simulink model "platforma3a"  (Simulink 8.3)
settings: Solver=ode23  StartTime=0.0  StopTime=80  RelTol=1e-8
values from neighbouring files (symbols this model uses):
  a = 0.365    [REX.m]
  b = 0.365    [REX.m]
  c = 0.387    [REX.m]
  d = 0.387    [REX.m]
  fr = 0    [REX.m]
  g = 9.81    [REX.m]
  Ik = 0.15    [REX.m]
  Ip = I    (= 6)    [REX.m]
  k1 = 1    [REX.m]
  k2 = 1    [REX.m]
  Kd = 500    [REX.m]
  mi = 0    [REX.m]
  mp = 40    [REX.m]
  omega = 0.1    [REX.m]
  R = 10    [REX.m]
  r = 0.127    [REX.m]
  tt = 0.387    [REX.m]
settings Model: Creator=mat  LastModifiedBy=Student
settings OptimizationCC: ExpressionDepthLimit=2147483647
settings DebuggingCC: FcnCallInpInsideContextMsg=UseLocalSettings

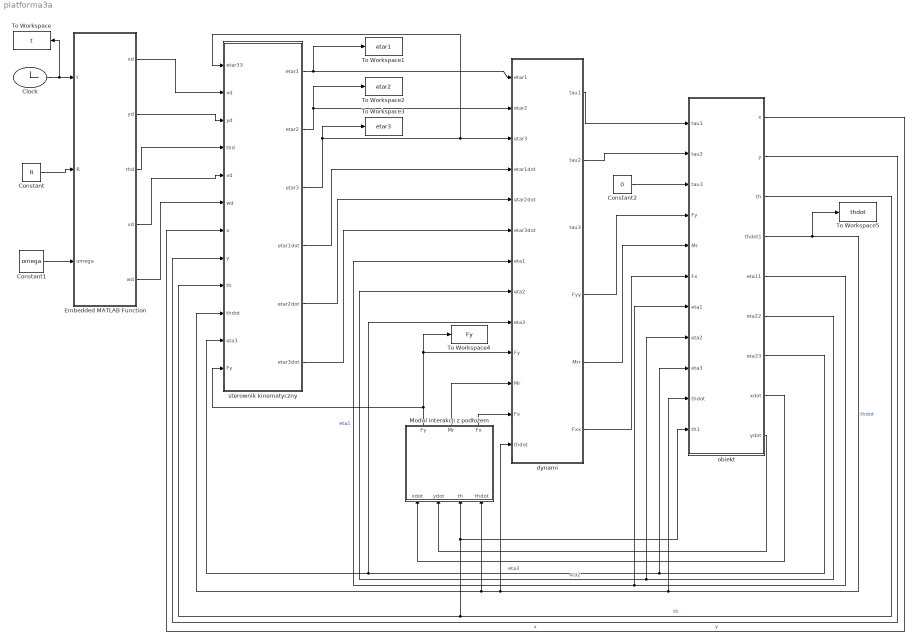
== system platforma3a ==
  Clock : Clock
  Constant : Constant  Value=R
  Constant1 : Constant  Value=omega
  Constant2 : Constant  Value=0
  Embedded MATLAB Function : MATLAB Function  TreatAsAtomicUnit=on
  Modul interakcji z podłożem : Subsystem
  To Workspace : ToWorkspace  VariableName=t  SampleTime=-1
  To Workspace1 : ToWorkspace  VariableName=etar1  SampleTime=-1
  To Workspace2 : ToWorkspace  VariableName=etar2  SampleTime=-1
  To Workspace3 : ToWorkspace  VariableName=etar3  SampleTime=-1
  To Workspace4 : ToWorkspace  VariableName=Fy  SampleTime=-1
  To Workspace5 : ToWorkspace  VariableName=thdot  SampleTime=-1
  dynami : Subsystem
  obiekt : Subsystem
  sterownik kinematyczny : Subsystem
  wires:
  Clock/1 -> Embedded MATLAB Function/1(t), To Workspace/1
  Constant/1 -> Embedded MATLAB Function/2(R)
  Constant1/1 -> Embedded MATLAB Function/3(omega)
  dynami/1(tau1) -> obiekt/1(tau1)
  dynami/2(tau2) -> obiekt/2(tau2)
  Modul interakcji z podłożem/3(Fx) -> dynami/12(Fx)
  dynami/4(Fyy) -> obiekt/4(Fy)
  dynami/5(Mrr) -> obiekt/5(Mr)
  dynami/6(Fxx) -> obiekt/6(Fx)
  obiekt/7(eta33) -> obiekt/9(eta3), dynami/9(eta3), sterownik kinematyczny/11(eta3)  "eta3"
  obiekt/6(eta22) -> obiekt/8(eta2), dynami/8(eta2)  "eta2"
  obiekt/5(eta11) -> obiekt/7(eta1), dynami/7(eta1)  "eta1"
  Embedded MATLAB Function/1(xd) -> sterownik kinematyczny/2(xd)
  Embedded MATLAB Function/2(yd) -> sterownik kinematyczny/3(yd)
  Embedded MATLAB Function/4(vd) -> sterownik kinematyczny/5(vd)
  Embedded MATLAB Function/5(wd) -> sterownik kinematyczny/6(wd)
  sterownik kinematyczny/1(etar1) -> dynami/1(etar1), To Workspace1/1
  sterownik kinematyczny/2(etar2) -> dynami/2(etar2), To Workspace2/1
  sterownik kinematyczny/3(etar3) -> To Workspace3/1, dynami/3(etar3), sterownik kinematyczny/1(etar33)
  sterownik kinematyczny/4(etar1dot) -> dynami/4(etar1dot)
  sterownik kinematyczny/5(etar2dot) -> dynami/5(etar2dot)
  sterownik kinematyczny/6(etar3dot) -> dynami/6(etar3dot)
  Modul interakcji z podłożem/2(Mr) -> dynami/11(Mr)
  Modul interakcji z podłożem/1(Fy) -> sterownik kinematyczny/12(Fy), dynami/10(Fy), To Workspace4/1
  obiekt/1(x) -> sterownik kinematyczny/7(x)  "x"
  obiekt/2(y) -> sterownik kinematyczny/8(y)  "y"
  obiekt/3(th) -> sterownik kinematyczny/9(th), Modul interakcji z podłożem/3(th), obiekt/11(th1)  "th"
  obiekt/4(thdot1) -> dynami/13(thdot), Modul interakcji z podłożem/4(thdot), sterownik kinematyczny/10(thdot), obiekt/10(thdot), To Workspace5/1  "thdot"
  obiekt/9(ydot) -> Modul interakcji z podłożem/2(ydot)
  obiekt/8(xdot) -> Modul interakcji z podłożem/1(xdot)
  Embedded MATLAB Function/3(thd) -> sterownik kinematyczny/4(thd)
  Constant2/1 -> obiekt/3(tau3)

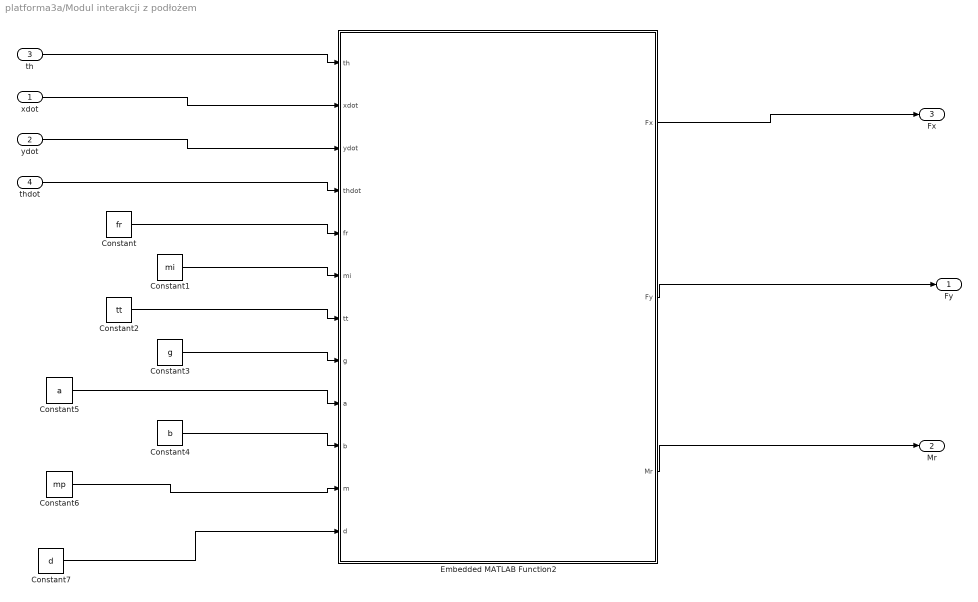
== system platforma3a/Modul interakcji z podłożem ==
  xdot : Inport
  ydot : Inport  Port=2
  th : Inport  Port=3
  thdot : Inport  Port=4
  Constant : Constant  Value=fr
  Constant1 : Constant  Value=mi
  Constant2 : Constant  Value=tt
  Constant3 : Constant  Value=g
  Constant4 : Constant  Value=b
  Constant5 : Constant  Value=a
  Constant6 : Constant  Value=mp
  Constant7 : Constant  Value=d
  Embedded MATLAB Function2 : MATLAB Function  TreatAsAtomicUnit=on
  Fy : Outport
  Mr : Outport  Port=2
  Fx : Outport  Port=3
  wires:
  th/1 -> Embedded MATLAB Function2/1(th)
  thdot/1 -> Embedded MATLAB Function2/4(thdot)
  Constant/1 -> Embedded MATLAB Function2/5(fr)
  Constant1/1 -> Embedded MATLAB Function2/6(mi)
  Constant2/1 -> Embedded MATLAB Function2/7(tt)
  Constant3/1 -> Embedded MATLAB Function2/8(g)
  Constant5/1 -> Embedded MATLAB Function2/9(a)
  Constant4/1 -> Embedded MATLAB Function2/10(b)
  Constant6/1 -> Embedded MATLAB Function2/11(m)
  Constant7/1 -> Embedded MATLAB Function2/12(d)
  Embedded MATLAB Function2/3(Mr) -> Mr/1
  Embedded MATLAB Function2/2(Fy) -> Fy/1
  Embedded MATLAB Function2/1(Fx) -> Fx/1
  xdot/1 -> Embedded MATLAB Function2/2(xdot)
  ydot/1 -> Embedded MATLAB Function2/3(ydot)

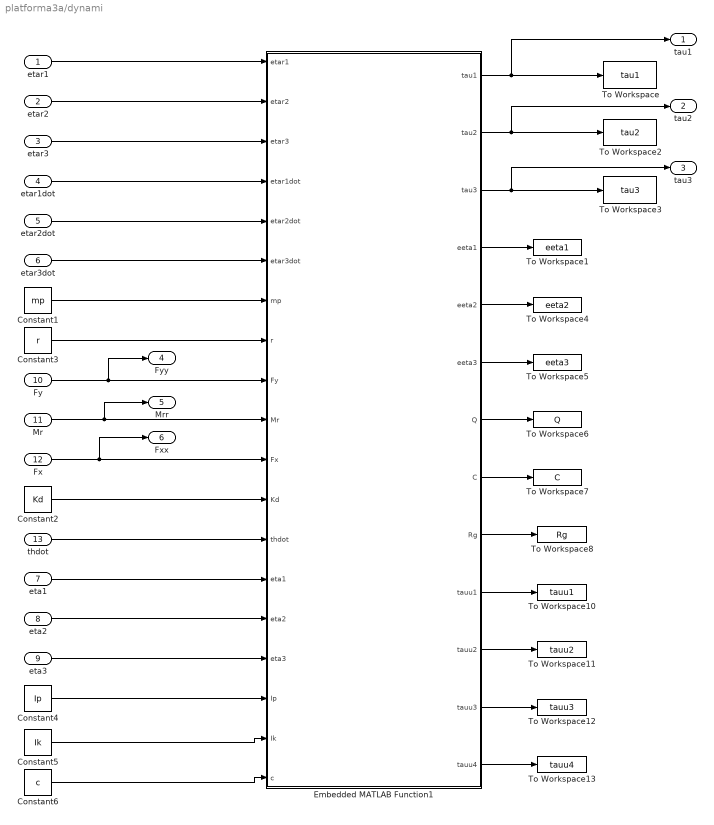
== system platforma3a/dynami ==
  etar1 : Inport
  etar2 : Inport  Port=2
  etar3 : Inport  Port=3
  etar1dot : Inport  Port=4
  etar2dot : Inport  Port=5
  etar3dot : Inport  Port=6
  eta1 : Inport  Port=7
  eta2 : Inport  Port=8
  eta3 : Inport  Port=9
  Fy : Inport  Port=10
  Mr : Inport  Port=11
  Fx : Inport  Port=12
  thdot : Inport  Port=13
  Constant1 : Constant  Value=mp
  Constant2 : Constant  Value=Kd
  Constant3 : Constant  Value=r
  Constant4 : Constant  Value=Ip
  Constant5 : Constant  Value=Ik
  Constant6 : Constant  Value=c
  Embedded MATLAB Function1 : MATLAB Function  TreatAsAtomicUnit=on
  To Workspace : ToWorkspace  VariableName=tau1  SampleTime=-1
  To Workspace1 : ToWorkspace  VariableName=eeta1  SampleTime=-1
  To Workspace10 : ToWorkspace  VariableName=tauu1  SampleTime=-1
  To Workspace11 : ToWorkspace  VariableName=tauu2  SampleTime=-1
  To Workspace12 : ToWorkspace  VariableName=tauu3  SampleTime=-1
  To Workspace13 : ToWorkspace  VariableName=tauu4  SampleTime=-1
  To Workspace2 : ToWorkspace  VariableName=tau2  SampleTime=-1
  To Workspace3 : ToWorkspace  VariableName=tau3  SampleTime=-1
  To Workspace4 : ToWorkspace  VariableName=eeta2  SampleTime=-1
  To Workspace5 : ToWorkspace  VariableName=eeta3  SampleTime=-1
  To Workspace6 : ToWorkspace  VariableName=Q  SampleTime=-1
  To Workspace7 : ToWorkspace  VariableName=C  SampleTime=-1
  To Workspace8 : ToWorkspace  VariableName=Rg  SampleTime=-1
  tau1 : Outport
  tau2 : Outport  Port=2
  tau3 : Outport  Port=3
  Fyy : Outport  Port=4
  Mrr : Outport  Port=5
  Fxx : Outport  Port=6
  wires:
  etar1/1 -> Embedded MATLAB Function1/1(etar1)
  etar2/1 -> Embedded MATLAB Function1/2(etar2)
  Embedded MATLAB Function1/1(tau1) -> tau1/1, To Workspace/1
  Embedded MATLAB Function1/2(tau2) -> To Workspace2/1, tau2/1
  Embedded MATLAB Function1/6(eeta3) -> To Workspace5/1
  Embedded MATLAB Function1/4(eeta1) -> To Workspace1/1
  Embedded MATLAB Function1/5(eeta2) -> To Workspace4/1
  Embedded MATLAB Function1/7(Q) -> To Workspace6/1
  Embedded MATLAB Function1/8(C) -> To Workspace7/1
  Embedded MATLAB Function1/9(Rg) -> To Workspace8/1
  Constant5/1 -> Embedded MATLAB Function1/18(Ik)
  Constant4/1 -> Embedded MATLAB Function1/17(Ip)
  eta3/1 -> Embedded MATLAB Function1/16(eta3)
  eta2/1 -> Embedded MATLAB Function1/15(eta2)
  eta1/1 -> Embedded MATLAB Function1/14(eta1)
  thdot/1 -> Embedded MATLAB Function1/13(thdot)
  Constant2/1 -> Embedded MATLAB Function1/12(Kd)
  Constant3/1 -> Embedded MATLAB Function1/8(r)
  Constant1/1 -> Embedded MATLAB Function1/7(mp)
  etar3dot/1 -> Embedded MATLAB Function1/6(etar3dot)
  etar2dot/1 -> Embedded MATLAB Function1/5(etar2dot)
  etar1dot/1 -> Embedded MATLAB Function1/4(etar1dot)
  etar3/1 -> Embedded MATLAB Function1/3(etar3)
  Embedded MATLAB Function1/13(tauu4) -> To Workspace13/1
  Embedded MATLAB Function1/12(tauu3) -> To Workspace12/1
  Embedded MATLAB Function1/11(tauu2) -> To Workspace11/1
  Embedded MATLAB Function1/10(tauu1) -> To Workspace10/1
  Constant6/1 -> Embedded MATLAB Function1/19(c)
  Fy/1 -> Embedded MATLAB Function1/9(Fy), Fyy/1
  Mr/1 -> Embedded MATLAB Function1/10(Mr), Mrr/1
  Fx/1 -> Embedded MATLAB Function1/11(Fx), Fxx/1
  Embedded MATLAB Function1/3(tau3) -> To Workspace3/1, tau3/1

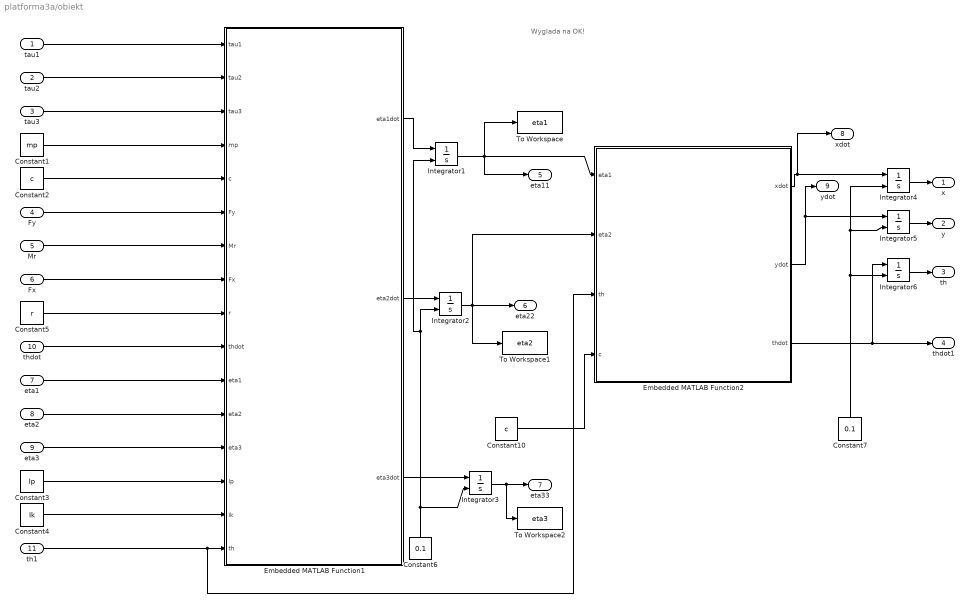
== system platforma3a/obiekt ==
  note: Wyglada na OK!
  tau1 : Inport
  tau2 : Inport  Port=2
  tau3 : Inport  Port=3
  Fy : Inport  Port=4
  Mr : Inport  Port=5
  Fx : Inport  Port=6
  eta1 : Inport  Port=7
  eta2 : Inport  Port=8
  eta3 : Inport  Port=9
  thdot : Inport  Port=10
  th1 : Inport  Port=11
  Constant1 : Constant  Value=mp
  Constant10 : Constant  Value=c
  Constant2 : Constant  Value=c
  Constant3 : Constant  Value=Ip
  Constant4 : Constant  Value=Ik
  Constant5 : Constant  Value=r
  Constant6 : Constant  Value=0.1
  Constant7 : Constant  Value=0.1
  Embedded MATLAB Function1 : MATLAB Function  TreatAsAtomicUnit=on
  Embedded MATLAB Function2 : MATLAB Function  TreatAsAtomicUnit=on
  Integrator{1..6} (6 alike) : Integrator  InitialConditionSource=external
  To Workspace : ToWorkspace  VariableName=eta1  SampleTime=-1
  To Workspace1 : ToWorkspace  VariableName=eta2  SampleTime=-1
  To Workspace2 : ToWorkspace  VariableName=eta3  SampleTime=-1
  x : Outport
  y : Outport  Port=2
  th : Outport  Port=3
  thdot1 : Outport  Port=4
  eta11 : Outport  Port=5
  eta22 : Outport  Port=6
  eta33 : Outport  Port=7
  xdot : Outport  Port=8
  ydot : Outport  Port=9
  wires:
  Constant1/1 -> Embedded MATLAB Function1/4(mp)
  Fy/1 -> Embedded MATLAB Function1/6(Fy)
  Mr/1 -> Embedded MATLAB Function1/7(Mr)
  tau1/1 -> Embedded MATLAB Function1/1(tau1)
  tau3/1 -> Embedded MATLAB Function1/3(tau3)
  tau2/1 -> Embedded MATLAB Function1/2(tau2)
  eta3/1 -> Embedded MATLAB Function1/13(eta3)
  eta1/1 -> Embedded MATLAB Function1/11(eta1)
  eta2/1 -> Embedded MATLAB Function1/12(eta2)
  thdot/1 -> Embedded MATLAB Function1/10(thdot)
  Fx/1 -> Embedded MATLAB Function1/8(Fx)
  Constant5/1 -> Embedded MATLAB Function1/9(r)
  Embedded MATLAB Function1/3(eta3dot) -> Integrator3/1
  Embedded MATLAB Function1/2(eta2dot) -> Integrator2/1
  Embedded MATLAB Function1/1(eta1dot) -> Integrator1/1
  Constant2/1 -> Embedded MATLAB Function1/5(c)
  Constant3/1 -> Embedded MATLAB Function1/14(Ip)
  Constant4/1 -> Embedded MATLAB Function1/15(Ik)
  Constant6/1 -> Integrator1/2, Integrator2/2, Integrator3/2
  Integrator3/1 -> eta33/1, To Workspace2/1
  Embedded MATLAB Function2/1(xdot) -> Integrator4/1, xdot/1
  Integrator4/1 -> x/1
  Integrator5/1 -> y/1
  Embedded MATLAB Function2/2(ydot) -> Integrator5/1, ydot/1
  Integrator6/1 -> th/1
  Constant7/1 -> Integrator4/2, Integrator5/2, Integrator6/2
  th1/1 -> Embedded MATLAB Function1/16(th), Embedded MATLAB Function2/3(th)
  Integrator1/1 -> To Workspace/1, eta11/1, Embedded MATLAB Function2/1(eta1)
  Integrator2/1 -> To Workspace1/1, Embedded MATLAB Function2/2(eta2), eta22/1
  Constant10/1 -> Embedded MATLAB Function2/4(c)
  Embedded MATLAB Function2/3(thdot) -> thdot1/1, Integrator6/1

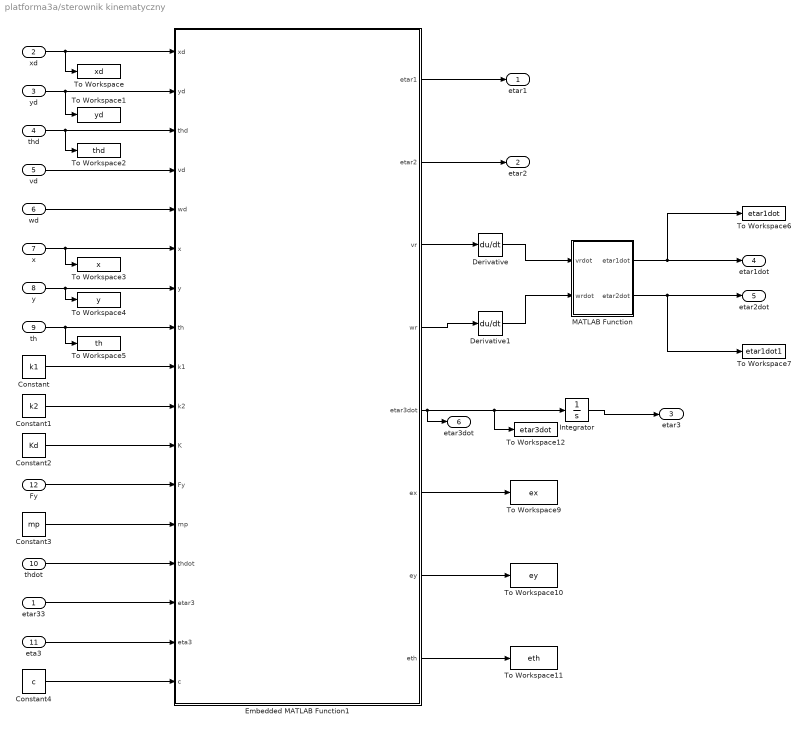
== system platforma3a/sterownik kinematyczny ==
  etar33 : Inport
  xd : Inport  Port=2
  yd : Inport  Port=3
  thd : Inport  Port=4
  vd : Inport  Port=5
  wd : Inport  Port=6
  x : Inport  Port=7
  y : Inport  Port=8
  th : Inport  Port=9
  thdot : Inport  Port=10
  eta3 : Inport  Port=11
  Fy : Inport  Port=12
  Constant : Constant  Value=k1
  Constant1 : Constant  Value=k2
  Constant2 : Constant  Value=Kd
  Constant3 : Constant  Value=mp
  Constant4 : Constant  Value=c
  Derivative : Derivative
  Derivative1 : Derivative
  Embedded MATLAB Function1 : MATLAB Function  TreatAsAtomicUnit=on
  Integrator : Integrator  InitialCondition=0.1
  MATLAB Function : MATLAB Function  TreatAsAtomicUnit=on
  To Workspace : ToWorkspace  VariableName=xd  SampleTime=-1
  To Workspace1 : ToWorkspace  VariableName=yd  SampleTime=-1
  To Workspace10 : ToWorkspace  VariableName=ey  SampleTime=-1
  To Workspace11 : ToWorkspace  VariableName=eth  SampleTime=-1
  To Workspace12 : ToWorkspace  VariableName=etar3dot  SampleTime=-1
  To Workspace2 : ToWorkspace  VariableName=thd  SampleTime=-1
  To Workspace3 : ToWorkspace  VariableName=x  SampleTime=-1
  To Workspace4 : ToWorkspace  VariableName=y  SampleTime=-1
  To Workspace5 : ToWorkspace  VariableName=th  SampleTime=-1
  To Workspace6 : ToWorkspace  VariableName=etar1dot  SampleTime=-1
  To Workspace7 : ToWorkspace  VariableName=etar1dot1  SampleTime=-1
  To Workspace9 : ToWorkspace  VariableName=ex  SampleTime=-1
  etar1 : Outport
  etar2 : Outport  Port=2
  etar3 : Outport  Port=3
  etar1dot : Outport  Port=4
  etar2dot : Outport  Port=5
  etar3dot : Outport  Port=6
  wires:
  Embedded MATLAB Function1/1(etar1) -> etar1/1
  Embedded MATLAB Function1/2(etar2) -> etar2/1
  Embedded MATLAB Function1/3(vr) -> Derivative/1
  Embedded MATLAB Function1/4(wr) -> Derivative1/1
  Derivative/1 -> MATLAB Function/1(vrdot)
  Derivative1/1 -> MATLAB Function/2(wrdot)
  MATLAB Function/1(etar1dot) -> etar1dot/1, To Workspace6/1
  MATLAB Function/2(etar2dot) -> etar2dot/1, To Workspace7/1
  Embedded MATLAB Function1/6(ex) -> To Workspace9/1
  Embedded MATLAB Function1/7(ey) -> To Workspace10/1
  Embedded MATLAB Function1/8(eth) -> To Workspace11/1
  xd/1 -> Embedded MATLAB Function1/1(xd), To Workspace/1
  yd/1 -> Embedded MATLAB Function1/2(yd), To Workspace1/1
  thd/1 -> Embedded MATLAB Function1/3(thd), To Workspace2/1
  vd/1 -> Embedded MATLAB Function1/4(vd)
  wd/1 -> Embedded MATLAB Function1/5(wd)
  x/1 -> Embedded MATLAB Function1/6(x), To Workspace3/1
  y/1 -> Embedded MATLAB Function1/7(y), To Workspace4/1
  th/1 -> Embedded MATLAB Function1/8(th), To Workspace5/1
  Constant/1 -> Embedded MATLAB Function1/9(k1)
  Constant1/1 -> Embedded MATLAB Function1/10(k2)
  Constant2/1 -> Embedded MATLAB Function1/11(K)
  Fy/1 -> Embedded MATLAB Function1/12(Fy)
  Constant3/1 -> Embedded MATLAB Function1/13(mp)
  thdot/1 -> Embedded MATLAB Function1/14(thdot)
  etar33/1 -> Embedded MATLAB Function1/15(etar3)
  eta3/1 -> Embedded MATLAB Function1/16(eta3)
  Constant4/1 -> Embedded MATLAB Function1/17(c)
  Embedded MATLAB Function1/5(etar3dot) -> etar3dot/1, Integrator/1, To Workspace12/1
  Integrator/1 -> etar3/1

== matlab function dynami/Embedded MATLAB Function1 ==
  data: etar1 input double; etar2 input double; tau1 output double; tau2 output double; tau3 output double; eeta1 output double; eeta2 output double; eeta3 output double; Q output double; C output double; Rg output double; etar3 input double; etar1dot input double; etar2dot input double; etar3dot input double; mp input double; r input double; Fy input double; Mr input double; Fx input double; Kd input double; thdot input double; eta1 input double; eta2 input double; eta3 input double; Ip input double; Ik input double; tauu1 output double; tauu2 output double; tauu3 output double; tauu4 output double; c input double
function [tau1,tau2,tau3, eeta1,eeta2,eeta3, Q, C, Rg,...
    tauu1, tauu2, tauu3, tauu4]  =fcn(etar1, etar2,...
etar3, etar1dot, etar2dot, etar3dot, mp,r, Fy,Mr, Fx,Kd, thdot,...
eta1,eta2,eta3,Ip, Ik, c)

%c=0.31;
tau=zeros(3,1);

eeta1=eta1-etar1;
eeta2=eta2-etar2;
eeta3=eta3-etar3;

invB =[r/2 0 0;
       0 r/2 0;
       0 0 1];
   
Q=[mp+Ip/c^2+4*Ik/r^2 mp-1/c^2*Ip 0;
   mp-1/c^2*Ip mp+Ip/c^2+4*Ik/r^2 0;
   0 0 mp];

C=[0 0 -mp*thdot;
   0 0 -mp*thdot;
   mp*thdot mp*thdot 0];
  

Rg=[-Fx-Mr/c;-Fx+Mr/c;-Fy];

en = [ eta1-etar1 ; eta2-etar2; eta3-etar3; ];
etar = [ etar1 ; etar2 ; etar3 ];
etardot = [etar1dot ; etar2dot ; etar3dot ];
tauu1 = invB * Q*etardot;
tauu2 = invB * C*etar;
tauu3 = invB * Rg;
tauu4 = invB * Kd*en;
tau=tauu1+tauu2+tauu3-tauu4;

tau1=tau(1,1);
tau2=tau(2,1);
tau3=tau(3,1);

== matlab function Embedded MATLAB Function ==
  data: xd output double; yd output double; thd output double; vd output double; wd output double; t input double; R input double; omega input double
 function [ xd, yd, thd,  vd, wd] = generator(t, R, omega)
% This block supports the Embedded MATLAB subset.
% See the help menu for details. 

xd=R*sin(omega*t);
yd=-R*cos(omega*t);
thd=omega*t;


 vd=1;
 wd=omega;

== matlab function obiekt/Embedded MATLAB Function1 ==
  data: tau1 input double; tau2 input double; tau3 input double; mp input double; c input double; Fy input double; Mr input double; Fx input double; r input double; thdot input double; eta1 input double; eta1dot output double; eta2dot output double; eta3dot output double; eta2 input double; eta3 input double; Ip input double; Ik input double; th input double
function [eta1dot,eta2dot,eta3dot]    =fcn(tau1, tau2, tau3, mp, c, Fy, Mr, Fx, r, thdot,...
    eta1,eta2,eta3, Ip, Ik, th)
%c=0.31;
etadot=zeros(3,1);
qdot=zeros(3,1);

B =[2/r 0 0;
    0 2/r 0;
    0 0 1];

M=[mp+Ip/c^2+4*Ik/r^2 mp-1/c^2*Ip 0;
   mp-1/c^2*Ip mp+Ip/c^2+4*Ik/r^2 0;
   0 0 mp];

C=[0 0 -mp*thdot;
   0 0 -mp*thdot;
   mp*thdot mp*thdot 0];
    
Rg=[-Fx-Mr/c;-Fx+Mr/c;-Fy];

tau = [ tau1 ; tau2 ; tau3 ];
eta = [ eta1 ; eta2 ; eta3 ];

etadot = inv(M) * (B*tau - C*eta - Rg);

eta1dot=etadot(1,1);
eta2dot=etadot(2,1);
eta3dot=etadot(3,1);

== matlab function Modul interakcji z podłożem/Embedded MATLAB Function2 ==
  data: th input double; xdot input double; ydot input double; Fx output double; thdot input double; fr input double; mi input double; tt input double; g input double; Fy output double; Mr output double; a input double; b input double; m input double; d input double
function [Fx, Fy, Mr] = fcn(th, xdot, ydot, thdot, fr, mi, tt, g,a,b, m, d)
%#eml

R=[cos(th) -sin(th);
    sin(th) cos(th)];

xx=inv(R)*[xdot; ydot];
% xx=[xdot; ydot];

x1p=xx(1,1)-tt*thdot;
x2p=xx(1,1)+tt*thdot;

y1p=xx(2,1)+a*thdot;
y3p=xx(2,1)-b*thdot;

Fx=fr*m*g*(sign(x1p)+sign(x2p))/2;
Fy=mi*m*g*(b*sign(y1p)+a*sign(y3p))/(a+b);
Mr=mi*a*b*m*g*(sign(y1p)-sign(y3p))/(a+b) + fr*tt*m*g*(sign(x2p)-sign(x1p))/2;

== matlab function sterownik kinematyczny/MATLAB Function ==
  data: vrdot input double; etar1dot output double; wrdot input double; etar2dot output double
function [etar1dot, etar2dot] = fcn(vrdot, wrdot)
%#codegen
L=0.31;
etar1dot=(vrdot-L*wrdot)/2;
etar2dot=(vrdot+L*wrdot)/2;

== matlab function sterownik kinematyczny/Embedded MATLAB Function1 ==
  data: xd input double; yd input double; thd input double; vd input double; wd input double; x input double; y input double; th input double; k1 input double; etar1 output double; etar2 output double; vr output double; wr output double; k2 input double; etar3dot output double; K input double; Fy input double; mp input double; thdot input double; etar3 input double; eta3 input double; ex output double; ey output double; eth output double; c input double
    function [etar1,etar2, vr, wr, etar3dot, ex,ey,eth] =fcn(xd,yd,thd,vd,wd,x,y,th,k1,k2, K, Fy, mp, thdot, etar3, eta3, c)
%L=0.31;
ex=xd-x;
ey=yd-y;
eth=thd-th;

xe=cos(th)*ex+sin(th)*ey;
ye=-sin(th)*ex+cos(th)*ey;
the=eth;

vr = k1*xe + vd*cos(the);
wr = wd + k2*the + vd*ye*sin(the)/the;
eeta3=eta3-etar3;

etar1 = (vr - c*wr)/2;
etar2 = (vr + c*wr)/2;

etar3dot=(K*eeta3+Fy-mp*thdot*(etar1+etar2))/mp;

== matlab function obiekt/Embedded MATLAB Function2 ==
  data: eta1 input double; xdot output double; ydot output double; thdot output double; eta2 input double; th input double; c input double
function [xdot,ydot,thdot]   =fcn(eta1,eta2,th, c)
%c=0.31;
L=c;

qdot=zeros(3,1);

G=[cos(th) cos(th);
    sin(th) sin(th);
    -1/c 1/c];

qdot=G*[eta1;eta2];

xdot=qdot(1,1);
ydot=qdot(2,1);
thdot=qdot(3,1);
